simulink model "guanxing3"  (R2023a)
settings: Solver=VariableStepAuto  StartTime=0.0  StopTime=0.005  RelTol=1e-3
settings Model: Creator=19405  LastModifiedBy=19405

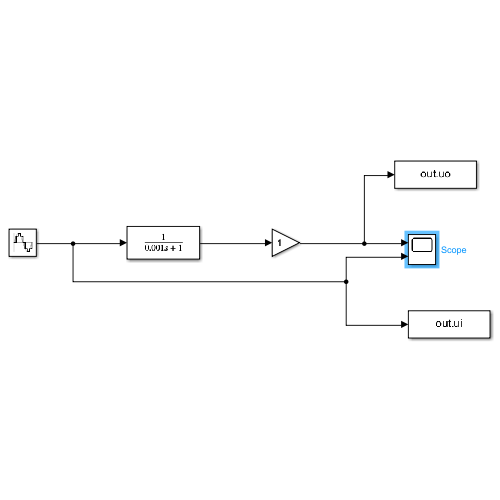
[thumbnail: Simulink's stored preview of the top-level diagram]
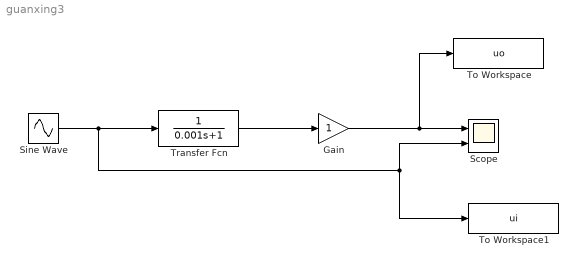
== system guanxing3 ==
  Gain : Gain
  Scope : Scope  NumInputPorts=2
  Sine Wave : Sin  Frequency=1884.95559  SampleTime=0.00001
  To Workspace : ToWorkspace  VariableName=uo  SaveFormat=Timeseries  SampleTime=-1
  To Workspace1 : ToWorkspace  VariableName=ui  SaveFormat=Timeseries  SampleTime=-1
  Transfer Fcn : TransferFcn  Denominator=[0.001 1]
  wires:
  Sine Wave/1 -> To Workspace1/1, Scope/2, Transfer Fcn/1
  Transfer Fcn/1 -> Gain/1
  Gain/1 -> To Workspace/1, Scope/1
